simulink model "VCM20"  (R2021b)
settings: Solver=ode1  StartTime=0.0  StopTime=Inf  FixedStep=0.001  RelTol=1e-3
PostLoadFcn:
  | , if any(exist('dsrtsu_mdlpostloadfcn', 'file') ~= 0), dsrtsu_mdlpostloadfcn('Execute', bdroot); end,
values from neighbouring files (symbols this model uses):
  gear_f = 14.45    [VehicleParamsFEM20_Gear17.m]
  Rwf = 18*(25.4/1000)/2    (= 0.2286)    [VehicleParamsFEM20_Gear17.m]
libraries: rtican x6
(part 2 of 2)

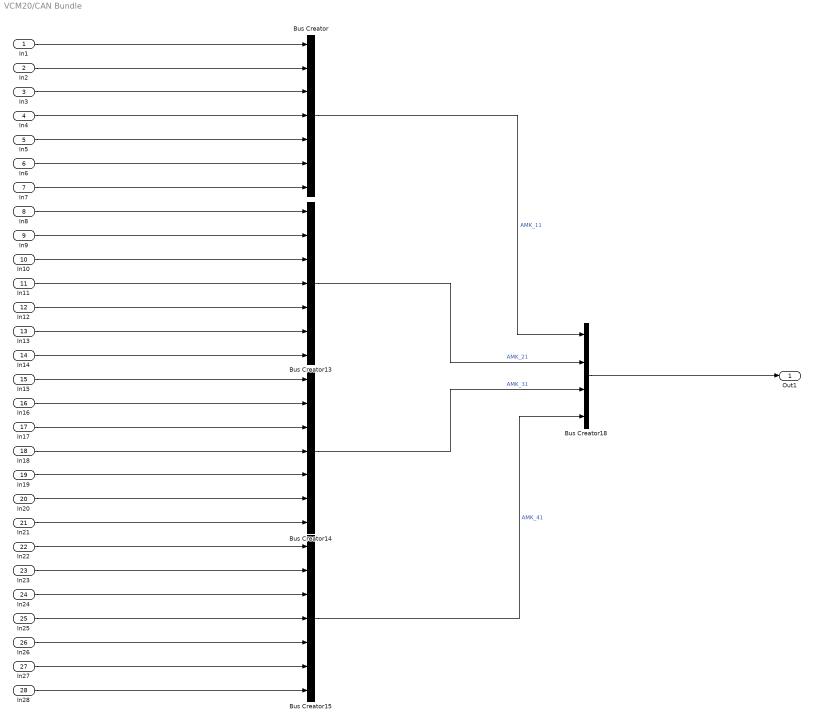
== system VCM20/CAN Bundle ==
  In1 : Inport
  In2 : Inport  Port=2
  In3 : Inport  Port=3
  In4 : Inport  Port=4
  In5 : Inport  Port=5
  In6 : Inport  Port=6
  In7 : Inport  Port=7
  In8 : Inport  Port=8
  In9 : Inport  Port=9
  In10 : Inport  Port=10
  In11 : Inport  Port=11
  In12 : Inport  Port=12
  In13 : Inport  Port=13
  In14 : Inport  Port=14
  In15 : Inport  Port=15
  In16 : Inport  Port=16
  In17 : Inport  Port=17
  In18 : Inport  Port=18
  In19 : Inport  Port=19
  In20 : Inport  Port=20
  In21 : Inport  Port=21
  In22 : Inport  Port=22
  In23 : Inport  Port=23
  In24 : Inport  Port=24
  In25 : Inport  Port=25
  In26 : Inport  Port=26
  In27 : Inport  Port=27
  In28 : Inport  Port=28
  Bus Creator{,13..15} (4 alike) : BusCreator  Inputs=7
  Bus Creator18 : BusCreator  Inputs=4
  Out1 : Outport  VectorParamsAs1DForOutWhenUnconnected=off
  wires:
  In12/1 -> Bus Creator13/5
  In16/1 -> Bus Creator14/2
  In24/1 -> Bus Creator15/3
  In10/1 -> Bus Creator13/3
  In9/1 -> Bus Creator13/2
  In15/1 -> Bus Creator14/1
  In20/1 -> Bus Creator14/6
  Bus Creator13/1 -> Bus Creator18/2  "AMK_21"
  In25/1 -> Bus Creator15/4
  In17/1 -> Bus Creator14/3
  Bus Creator15/1 -> Bus Creator18/4  "AMK_41"
  In21/1 -> Bus Creator14/7
  In14/1 -> Bus Creator13/7
  In23/1 -> Bus Creator15/2
  In27/1 -> Bus Creator15/6
  In26/1 -> Bus Creator15/5
  Bus Creator/1 -> Bus Creator18/1  "AMK_11"
  In11/1 -> Bus Creator13/4
  In22/1 -> Bus Creator15/1
  In19/1 -> Bus Creator14/5
  Bus Creator14/1 -> Bus Creator18/3  "AMK_31"
  In28/1 -> Bus Creator15/7
  In13/1 -> Bus Creator13/6
  In18/1 -> Bus Creator14/4
  In8/1 -> Bus Creator13/1
  In1/1 -> Bus Creator/1
  In2/1 -> Bus Creator/2
  In3/1 -> Bus Creator/3
  In4/1 -> Bus Creator/4
  In5/1 -> Bus Creator/5
  In6/1 -> Bus Creator/6
  In7/1 -> Bus Creator/7
  Bus Creator18/1 -> Out1/1

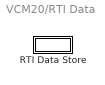
== system VCM20/RTI Data ==
  RTI Data Store : Subsystem  Tag="struct('private',struct('version',struct('dsVer',uint32(2)),'access',struct('modified',['01-Aug-2023 16:47:04'],'type','Model','isPerm',1)),'public',struct('main',struct('data',[]),'sub',struct('name',{{'VCM20'}},'data',{{struct('TH',struct('thTaskInfo',struct('taskType',{'TIMER','HWINT','TMRINT','SWINT','GLINT'},'tasksNumOf',{1,0,0,0,0},'srcIds',{{'TIMERA'},{},{},{},{}},'taskNames',{{['Timer Task 1']},{},{},{},{}})),'th_tc',struct('dataType','TASK','taskGroupId','','taskGroupList',{{}},'taskSchedulingPolicy','FCFS','taskType','TIMER','blkh',-1,'srcId','TIMERA','srcSgnName',['Timer A interrupt'],'srcCpuName','','taskName',['Timer Task 1  [0.001] s'],'taskNameDisplayExt','','smplTime',0.001,'smplTimeOffs',0,'hasFixedPriority',0,'priority',1,'hasFixedOvc',0,'ovcType',1,'ovcMax',1),'tc_th',struct('dataType','TASK','taskGroupId','','taskGroupList',{{}},'taskSchedulingPolicy','FCFS','taskType','TIMER','blkh',-1,'srcId','TIMERA','srcSgnName',['Timer A interrupt'],'srcCpuName','','taskName',['Timer Task 1  [0.001] s'],'taskNameDisplayExt','','smplTime',0.001,'smplTimeOffs',0,'hasFixedPriority',0,'priority',1,'hasFixedOvc',0,'ovcType',1,'ovcMax',1))}})))"  mask(RTI_DATA_STORE){}
      mask help:
      | RTI Data Store Block. This block is used by RTI to store internal model dependent data. Deleting this block will result in data loss.
      |
      | NEVER DELETE, COPY, OR MODIFY THIS BLOCK!
      mask Help:
      | RTI Data Store Block. This block is used by RTI to store internal model dependent data. Deleting this block will result in data loss.
      | 
      | NEVER DELETE, COPY, OR MODIFY THIS BLOCK!
      mask Display: text(0.5, 0.5, ' ', 'HorizontalAlignment', 'center');

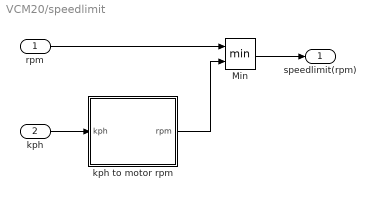
== system VCM20/speedlimit ==
  rpm : Inport
  kph : Inport  Port=2
  Min : MinMax  Inputs=2
  kph to motor rpm : Subsystem
  speedlimit(rpm) : Outport  VectorParamsAs1DForOutWhenUnconnected=off
  wires:
  kph/1 -> kph to motor rpm/1(kph)
  Min/1 -> speedlimit(rpm)/1
  rpm/1 -> Min/1
  kph to motor rpm/1(rpm) -> Min/2

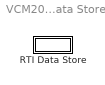
== system VCM20/RTI Data/RTI Data Store ==
  RTI Data Store : Subsystem  mask(RTI_DATA_STORE){}
      mask help:
      | RTI Data Store Block. This block is used by RTI to store internal model dependent data. Deleting this block will result in data loss.
      |
      | NEVER DELETE, COPY, OR MODIFY THIS BLOCK!
      mask Help:
      | RTI Data Store Block. This block is used by RTI to store internal model dependent data. Deleting this block will result in data loss.
      | 
      | NEVER DELETE, COPY, OR MODIFY THIS BLOCK!
      mask Display: text(0.5, 0.5, ' ', 'HorizontalAlignment', 'center');

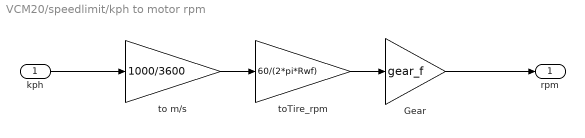
== system VCM20/speedlimit/kph to motor rpm ==
  kph : Inport
  Gear : Gain  Gain=gear_f
  to m/s : Gain  Gain=1000/3600
  toTire_rpm : Gain  Gain=60/(2*pi*Rwf)
  rpm : Outport  VectorParamsAs1DForOutWhenUnconnected=off
  wires:
  kph/1 -> to m/s/1
  toTire_rpm/1 -> Gear/1
  to m/s/1 -> toTire_rpm/1
  Gear/1 -> rpm/1

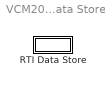
== system VCM20/RTI Data/RTI Data Store/RTI Data Store ==
  RTI Data Store : Subsystem  mask(RTI_DATA_STORE){}
      mask help:
      | RTI Data Store Block. This block is used by RTI to store internal model dependent data. Deleting this block will result in data loss.
      |
      | NEVER DELETE, COPY, OR MODIFY THIS BLOCK!
      mask Help:
      | RTI Data Store Block. This block is used by RTI to store internal model dependent data. Deleting this block will result in data loss.
      | 
      | NEVER DELETE, COPY, OR MODIFY THIS BLOCK!
      mask Display: text(0.5, 0.5, ' ', 'HorizontalAlignment', 'center');

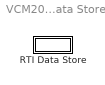
== system VCM20/RTI Data/RTI Data Store/RTI Data Store/RTI Data Store ==
  RTI Data Store : Subsystem  mask(RTI_DATA_STORE){}
      mask help:
      | RTI Data Store Block. This block is used by RTI to store internal model dependent data. Deleting this block will result in data loss.
      |
      | NEVER DELETE, COPY, OR MODIFY THIS BLOCK!
      mask Help:
      | RTI Data Store Block. This block is used by RTI to store internal model dependent data. Deleting this block will result in data loss.
      | 
      | NEVER DELETE, COPY, OR MODIFY THIS BLOCK!
      mask Display: text(0.5, 0.5, ' ', 'HorizontalAlignment', 'center');

== system VCM20/RTI Data/RTI Data Store/RTI Data Store/RTI Data Store/RTI Data Store ==
